simulink library "RxTxFixedPointLibrary"  (R2017b)
settings: Solver=VariableStepAuto  StartTime=0.0  StopTime=10.0  RelTol=1e-3
undefined symbols (not defined in the file): AGCBarkerSymbols, coeff, crcDecodeLag, CRCGeneratorLag, EQTrainingSymbols, j, K1, K2, numHeaderBits, numTrainingSamples, pLen, RadioSampleRate, samplesPerSymbol, VibertiTracebackLength, xPreambleSeq
libraries: simulink x27, dsphdlfiltering x20, hdlsllib x10, commseqgen3 x4, commdigbbndpm3 x3, commcrc2 x2, commcnvcod2 x2, dspsigops x2, dspstat3 x1, commfilt2 x1
(part 1 of 3)
settings Model: Creator=tcollins  LastModifiedBy=tcollins

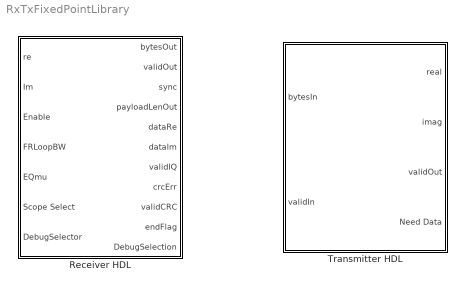
== system RxTxFixedPointLibrary ==
  Receiver HDL : Subsystem  TreatAsAtomicUnit=on
      mask Display:
      | if ispc
      |     d = '\';
      | else
      |     d = '/';
      | end
      | model_path = get_param(bdroot, 'FileName');
      | %info = Simulink.MDLInfo(bdroot)
      | c = strsplit(model_path,d); c = strjoin(c(1:end-2),d);
      | logo = [c,d,'ADI_logo.svg'];
      | %disp(logo);
      | image(logo);
  Transmitter HDL : Subsystem  TreatAsAtomicUnit=on
      mask Display:
      | if ispc
      |     d = '\';
      | else
      |     d = '/';
      | end
      | model_path = get_param(bdroot, 'FileName');
      | %info = Simulink.MDLInfo(bdroot)
      | c = strsplit(model_path,d); c = strjoin(c(1:end-2),d);
      | logo = [c,d,'ADI_logo.svg'];
      | %disp(logo);
      | image(logo);

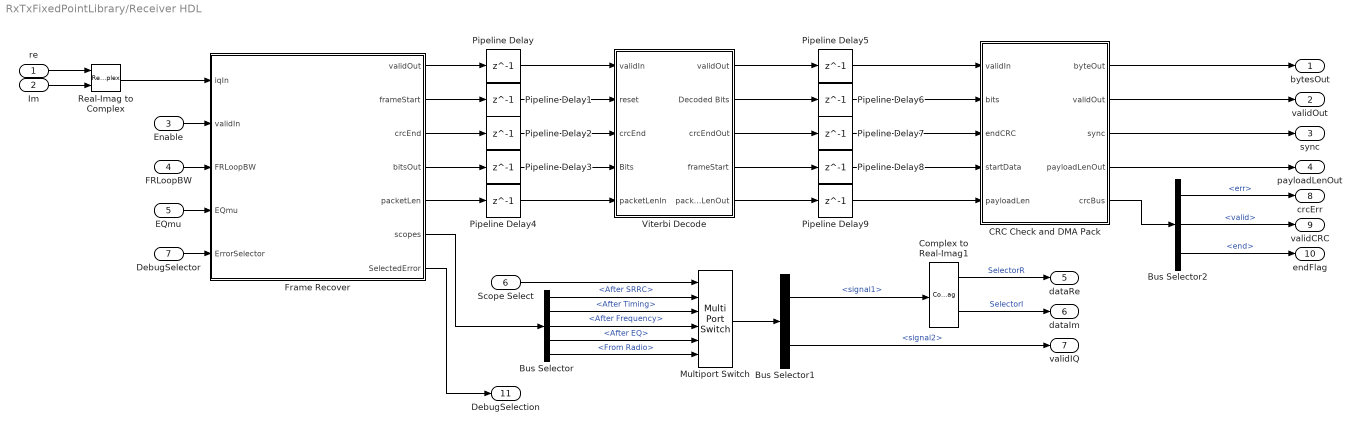
== system RxTxFixedPointLibrary/Receiver HDL ==
  re : Inport  OutDataTypeStr=int16
  Im : Inport  Port=2  OutDataTypeStr=int16
  Enable : Inport  Port=3
  FRLoopBW : Inport  Port=4
  EQmu : Inport  Port=5
  Scope Select : Inport  Port=6
  DebugSelector : Inport  Port=7
  Bus Selector : BusSelector  OutputSignals=After SRRC,After Timing,After Frequency,After EQ,From Radio
  Bus Selector1 : BusSelector  OutputSignals=signal1,signal2
  Bus Selector2 : BusSelector  OutputSignals=err,valid,end
  CRC Check and DMA Pack : Subsystem
  Complex to Real-Imag1 : ComplexToRealImag
  Frame Recover : Subsystem
  Multiport Switch : MultiPortSwitch  Inputs=5
  Pipeline Delay{,1..9} (10 alike) : Delay  DelayLength=1
  Real-Imag to Complex : RealImagToComplex
  Viterbi Decode : Subsystem  TreatAsAtomicUnit=on
  bytesOut : Outport
  validOut : Outport  Port=2
  sync : Outport  Port=3
  payloadLenOut : Outport  Port=4
  dataRe : Outport  Port=5
  dataIm : Outport  Port=6
  validIQ : Outport  Port=7
  crcErr : Outport  Port=8
  validCRC : Outport  Port=9
  endFlag : Outport  Port=10
  DebugSelection : Outport  Port=11
  wires:
  Bus Selector/5 -> Multiport Switch/6  "<From Radio>"
  Pipeline Delay5/1 -> CRC Check and DMA Pack/1(validIn)
  Bus Selector1/2 -> validIQ/1  "<signal2>"
  Bus Selector1/1 -> Complex to Real-Imag1/1  "<signal1>"
  Bus Selector/4 -> Multiport Switch/5  "<After EQ>"
  Multiport Switch/1 -> Bus Selector1/1
  Scope Select/1 -> Multiport Switch/1
  Bus Selector/2 -> Multiport Switch/3  "<After Timing>"
  Bus Selector/3 -> Multiport Switch/4  "<After Frequency>"
  Bus Selector/1 -> Multiport Switch/2  "<After SRRC>"
  Frame Recover/6(scopes) -> Bus Selector/1
  EQmu/1 -> Frame Recover/4(EQmu)
  FRLoopBW/1 -> Frame Recover/3(FRLoopBW)
  Viterbi Decode/1(validOut) -> Pipeline Delay5/1
  Pipeline Delay/1 -> Viterbi Decode/1(validIn)
  CRC Check and DMA Pack/4(payloadLenOut) -> payloadLenOut/1
  Viterbi Decode/2(Decoded Bits) -> Pipeline Delay6/1
  Pipeline Delay2/1 -> Viterbi Decode/3(crcEnd)
  CRC Check and DMA Pack/3(sync) -> sync/1
  Pipeline Delay7/1 -> CRC Check and DMA Pack/3(endCRC)
  Pipeline Delay9/1 -> CRC Check and DMA Pack/5(payloadLen)
  Pipeline Delay6/1 -> CRC Check and DMA Pack/2(bits)
  Pipeline Delay8/1 -> CRC Check and DMA Pack/4(startData)
  Pipeline Delay4/1 -> Viterbi Decode/5(packetLenIn)
  Pipeline Delay3/1 -> Viterbi Decode/4(Bits)
  Pipeline Delay1/1 -> Viterbi Decode/2(reset)
  CRC Check and DMA Pack/2(validOut) -> validOut/1
  CRC Check and DMA Pack/1(byteOut) -> bytesOut/1
  Viterbi Decode/5(packetLenOut) -> Pipeline Delay9/1
  Viterbi Decode/4(frameStart) -> Pipeline Delay8/1
  Viterbi Decode/3(crcEndOut) -> Pipeline Delay7/1
  Frame Recover/4(bitsOut) -> Pipeline Delay3/1
  Frame Recover/3(crcEnd) -> Pipeline Delay2/1
  Frame Recover/2(frameStart) -> Pipeline Delay1/1
  Frame Recover/1(validOut) -> Pipeline Delay/1
  Frame Recover/5(packetLen) -> Pipeline Delay4/1
  Complex to Real-Imag1/1 -> dataRe/1  "SelectorR"
  Complex to Real-Imag1/2 -> dataIm/1  "SelectorI"
  Im/1 -> Real-Imag to Complex/2
  re/1 -> Real-Imag to Complex/1
  CRC Check and DMA Pack/5(crcBus) -> Bus Selector2/1
  Bus Selector2/1 -> crcErr/1  "<err>"
  Bus Selector2/2 -> validCRC/1  "<valid>"
  Bus Selector2/3 -> endFlag/1  "<end>"
  Enable/1 -> Frame Recover/2(validIn)
  Real-Imag to Complex/1 -> Frame Recover/1(iqIn)
  DebugSelector/1 -> Frame Recover/5(ErrorSelector)
  Frame Recover/7(SelectedError) -> DebugSelection/1

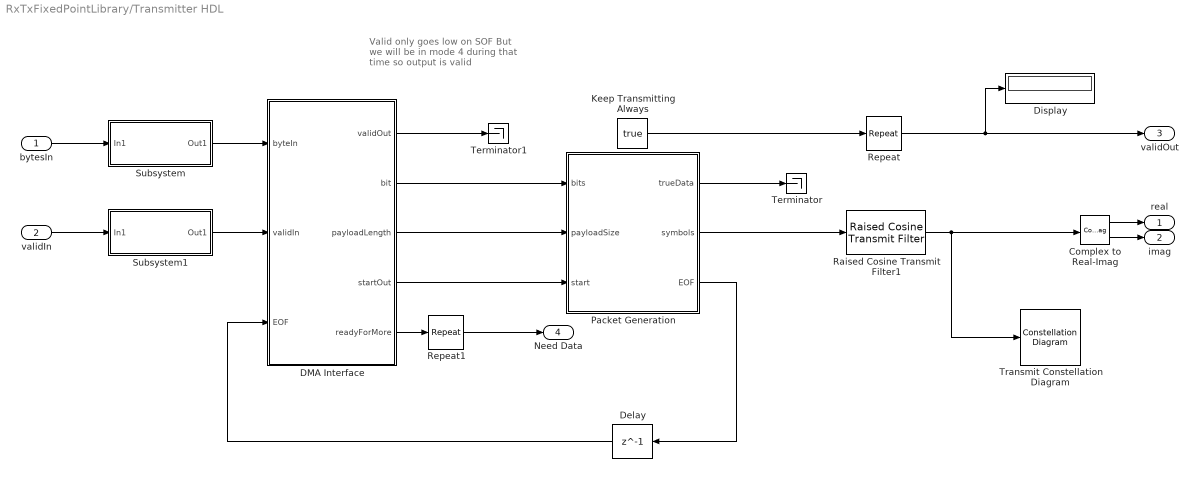
== system RxTxFixedPointLibrary/Transmitter HDL ==
  note: Valid only goes low on SOF
      | But we will be in mode 4 during
      | that time so output is valid
  bytesIn : Inport
  validIn : Inport  Port=2
  Complex to Real-Imag : ComplexToRealImag
  DMA Interface : Subsystem
  Delay : Delay  DelayLength=1
  Display : Display
  Keep Transmitting Always : Constant  Value=true  SampleTime=-1
  Packet Generation : Subsystem
  Raised Cosine Transmit Filter1 : commfilt2/Raised Cosine Transmit Filter  filtType=Square root  R=0.5  filtSpan=8  N=4  filterGain=1  RateOptions=Allow multirate processing  framing=Mute  checkCoeff=off  variableName=rcTxFilt1  checkGain=Normalized  sampMode=Mute  saveAsFlag=0  currentFiltSpan=8  D=(8)/2  launchFVT=on  roundingMode=Floor  overflowMode=off  coeffDataTypeStr=Inherit: Same word length as input  coeffMin=[]  coeffMax=[]  coeffLastDataTypeStr=Inherit: Same word length as input  outputMode=Binary point scaling  outputWordLength=16  outputFracLength=14  outputDataTypeStr=fixdt(1,16,14)  outputMin=[]  outputMax=[]  outputLastDataTypeStr=fixdt(1,16,14)
  Repeat : dspsigops/Repeat  N=4  InputProcessing=Columns as channels (frame based)  RateOptions=Allow multirate processing  ic=0  mode=Unused parameter value
      settings: SourceProductName=DSP System Toolbox
  Repeat1 : dspsigops/Repeat  N=4  InputProcessing=Columns as channels (frame based)  RateOptions=Allow multirate processing  ic=0  mode=Unused parameter value
      settings: SourceProductName=DSP System Toolbox
  Subsystem : Subsystem
  Subsystem1 : Subsystem
  Terminator : Terminator
  Terminator1 : Terminator
  Transmit Constellation Diagram : ConstellationDiagram
  real : Outport  PortDimensions=1
  imag : Outport  Port=2  PortDimensions=1
  validOut : Outport  Port=3  PortDimensions=1
  Need Data : Outport  Port=4
  wires:
  Complex to Real-Imag/1 -> real/1
  Complex to Real-Imag/2 -> imag/1
  DMA Interface/2(bit) -> Packet Generation/1(bits)
  DMA Interface/3(payloadLength) -> Packet Generation/2(payloadSize)
  DMA Interface/4(startOut) -> Packet Generation/3(start)
  Packet Generation/2(symbols) -> Raised Cosine Transmit Filter1/1
  DMA Interface/5(readyForMore) -> Repeat1/1
  Packet Generation/1(trueData) -> Terminator/1
  Packet Generation/3(EOF) -> Delay/1
  Delay/1 -> DMA Interface/3(EOF)
  bytesIn/1 -> Subsystem/1(In1)
  Repeat1/1 -> Need Data/1
  Subsystem/1(Out1) -> DMA Interface/1(byteIn)
  Subsystem1/1(Out1) -> DMA Interface/2(validIn)
  DMA Interface/1(validOut) -> Terminator1/1
  Keep Transmitting Always/1 -> Repeat/1
  validIn/1 -> Subsystem1/1(In1)
  Repeat/1 -> validOut/1, Display/1
  Raised Cosine Transmit Filter1/1 -> Transmit Constellation Diagram/1, Complex to Real-Imag/1

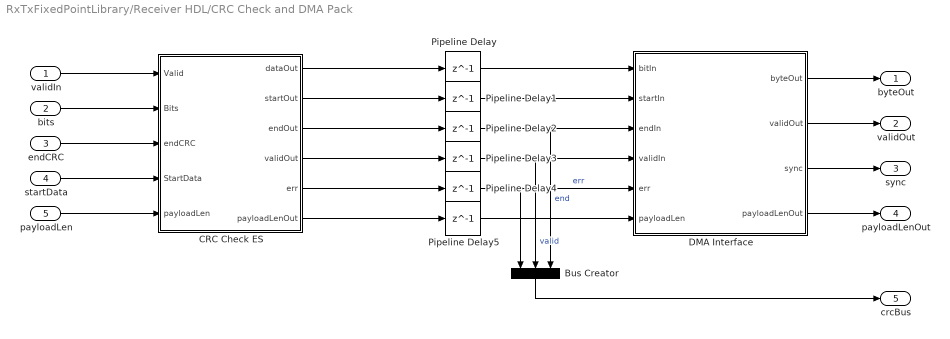
== system RxTxFixedPointLibrary/Receiver HDL/CRC Check and DMA Pack ==
  validIn : Inport  PortDimensions=1
  bits : Inport  Port=2  PortDimensions=1
  endCRC : Inport  Port=3  PortDimensions=1
  startData : Inport  Port=4  PortDimensions=1
  payloadLen : Inport  Port=5  PortDimensions=1
  Bus Creator : BusCreator  Inputs=3
  CRC Check ES : Subsystem
  DMA Interface : Subsystem
  Pipeline Delay{,1..5} (6 alike) : Delay  DelayLength=1
  byteOut : Outport
  validOut : Outport  Port=2
  sync : Outport  Port=3
  payloadLenOut : Outport  Port=4
  crcBus : Outport  Port=5
  wires:
  CRC Check ES/4(validOut) -> Pipeline Delay3/1
  DMA Interface/4(payloadLenOut) -> payloadLenOut/1
  validIn/1 -> CRC Check ES/1(Valid)
  Pipeline Delay5/1 -> DMA Interface/6(payloadLen)
  Pipeline Delay4/1 -> Bus Creator/1, DMA Interface/5(err)  "err"
  Pipeline Delay3/1 -> Bus Creator/2, DMA Interface/4(validIn)  "valid"
  Pipeline Delay2/1 -> Bus Creator/3, DMA Interface/3(endIn)  "end"
  Pipeline Delay1/1 -> DMA Interface/2(startIn)
  Pipeline Delay/1 -> DMA Interface/1(bitIn)
  endCRC/1 -> CRC Check ES/3(endCRC)
  CRC Check ES/6(payloadLenOut) -> Pipeline Delay5/1
  startData/1 -> CRC Check ES/4(StartData)
  payloadLen/1 -> CRC Check ES/5(payloadLen)
  DMA Interface/3(sync) -> sync/1
  bits/1 -> CRC Check ES/2(Bits)
  CRC Check ES/5(err) -> Pipeline Delay4/1
  CRC Check ES/1(dataOut) -> Pipeline Delay/1
  CRC Check ES/2(startOut) -> Pipeline Delay1/1
  DMA Interface/1(byteOut) -> byteOut/1
  CRC Check ES/3(endOut) -> Pipeline Delay2/1
  DMA Interface/2(validOut) -> validOut/1
  Bus Creator/1 -> crcBus/1

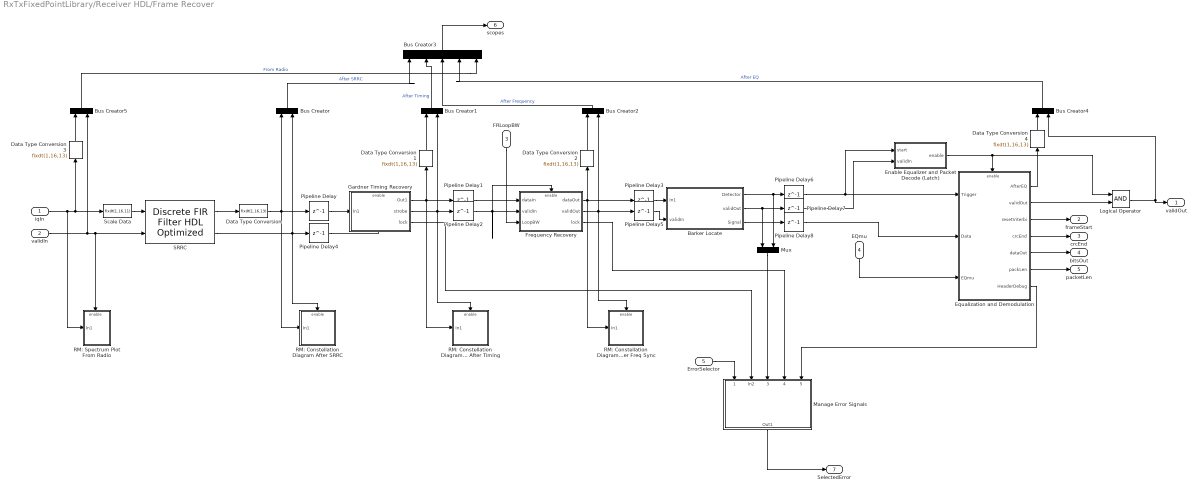
== system RxTxFixedPointLibrary/Receiver HDL/Frame Recover ==
  iqIn : Inport  PortDimensions=1
  validIn : Inport  Port=2  PortDimensions=1
  FRLoopBW : Inport  Port=3
  EQmu : Inport  Port=4
  ErrorSelector : Inport  Port=5  PortDimensions=1
  Barker Locate : Subsystem  mask{Threshold=1}
  Bus Creator{,1..2,4..5} (5 alike) : BusCreator  Inputs=2
  Bus Creator3 : BusCreator  Inputs=5
  Data Type Conversion{,1..4} (5 alike) : DataTypeConversion  OutDataTypeStr=fixdt(1,16,13)
  Enable Equalizer and Packet Decode (Latch) : MATLAB Function  TreatAsAtomicUnit=on
  Equalization and Demodulation : Subsystem
  Frequency Recovery : Subsystem
  Gardner Timing Recovery : Subsystem
  Logical Operator : Logic  AllPortsSameDT=off  OutDataTypeStr=boolean
  Manage Error Signals : Subsystem
  Mux : Mux  Inputs=2
  Pipeline Delay{,1..8} (9 alike) : Delay  DelayLength=1
  RM: Constellation Diagram After Freq Sync : Subsystem
  RM: Constellation Diagram After SRRC : Subsystem
  RM: Constellation Diagram After Timing : Subsystem
  RM: Spectrum Plot From Radio : Subsystem
  SRRC : dsphdlfiltering/Discrete FIR Filter HDL Optimized  Numerator=coeff  Sharing=off  SharingFactor=2  SimulateUsing=Code generation  roundingMode=Floor  overflowMode=on  CoefficientsDataTypeStr=Inherit: Same word length as input  CoefficientsMin=[]  CoefficientsMax=[]  OutputDataTypeStr=fixdt(1,16,11)  OutputMin=[]  OutputMax=[]  ValidInPort=on  ReadyPort=off
      settings: SourceProductName=DSP System Toolbox  SourceProductBaseCode=DS
  Scale Data : DataTypeConversion  OutDataTypeStr=fixdt(1,16,11)  ConvertRealWorld=Stored Integer (SI)  SaturateOnIntegerOverflow=on
  validOut : Outport
  frameStart : Outport  Port=2
  crcEnd : Outport  Port=3
  bitsOut : Outport  Port=4
  packetLen : Outport  Port=5
  scopes : Outport  Port=6
  SelectedError : Outport  Port=7
  wires:
  Data Type Conversion3/1 -> Bus Creator5/1
  Bus Creator5/1 -> Bus Creator3/5  "From Radio"
  Data Type Conversion4/1 -> Bus Creator4/1
  Data Type Conversion2/1 -> Bus Creator2/1
  Data Type Conversion1/1 -> Bus Creator1/1
  Bus Creator4/1 -> Bus Creator3/4  "After EQ"
  Bus Creator3/1 -> scopes/1
  Bus Creator2/1 -> Bus Creator3/3  "After Frequency"
  Bus Creator1/1 -> Bus Creator3/2  "After Timing"
  Bus Creator/1 -> Bus Creator3/1  "After SRRC"
  Frequency Recovery/2(validOut) -> RM: Constellation Diagram After Freq Sync/Enable, Bus Creator2/2, Pipeline Delay5/1
  Frequency Recovery/1(dataOut) -> Data Type Conversion2/1, RM: Constellation Diagram After Freq Sync/1(In1), Pipeline Delay3/1
  Gardner Timing Recovery/1(Out1) -> Pipeline Delay1/1, Data Type Conversion1/1, RM: Constellation Diagram After Timing/1(In1)
  Gardner Timing Recovery/2(strobe) -> RM: Constellation Diagram After Timing/Enable, Pipeline Delay2/1, Bus Creator1/2
  EQmu/1 -> Equalization and Demodulation/3(EQmu)
  FRLoopBW/1 -> Frequency Recovery/3(LoopBW)
  Pipeline Delay4/1 -> Gardner Timing Recovery/Enable
  Pipeline Delay/1 -> Gardner Timing Recovery/1(In1)
  Data Type Conversion/1 -> Bus Creator/1, Pipeline Delay/1, RM: Constellation Diagram After SRRC/1(In1)
  Logical Operator/1 -> validOut/1, Bus Creator4/2
  Pipeline Delay8/1 -> Equalization and Demodulation/2(Data)
  Pipeline Delay7/1 -> Enable Equalizer and Packet Decode (Latch)/2(validIn)
  Pipeline Delay6/1 -> Equalization and Demodulation/1(Trigger), Enable Equalizer and Packet Decode (Latch)/1(start)
  Pipeline Delay5/1 -> Barker Locate/2(validIn)
  Pipeline Delay3/1 -> Barker Locate/1(In1)
  Pipeline Delay2/1 -> Frequency Recovery/Enable, Frequency Recovery/2(validIn)
  Pipeline Delay1/1 -> Frequency Recovery/1(dataIn)
  Equalization and Demodulation/1(AfterEQ) -> Data Type Conversion4/1
  Barker Locate/1(Detector) -> Mux/2, Pipeline Delay6/1
  Equalization and Demodulation/6(packLen) -> packetLen/1
  Scale Data/1 -> SRRC/1
  Equalization and Demodulation/2(validOut) -> Logical Operator/2
  Barker Locate/3(Signal) -> Pipeline Delay8/1
  validIn/1 -> Bus Creator5/2, RM: Spectrum Plot From Radio/Enable, SRRC/2
  iqIn/1 -> RM: Spectrum Plot From Radio/1(In1), Data Type Conversion3/1, Scale Data/1
  SRRC/1 -> Data Type Conversion/1
  SRRC/2 -> Bus Creator/2, Pipeline Delay4/1, RM: Constellation Diagram After SRRC/Enable
  Equalization and Demodulation/5(dataOut) -> bitsOut/1
  Enable Equalizer and Packet Decode (Latch)/1(enable) -> Equalization and Demodulation/Enable, Logical Operator/1
  Equalization and Demodulation/4(crcEnd) -> crcEnd/1
  Barker Locate/2(validOut) -> Mux/1, Pipeline Delay7/1
  Equalization and Demodulation/3(resetViterbi) -> frameStart/1
  Mux/1 -> Manage Error Signals/3(Peak Detector)
  Frequency Recovery/3(lock) -> Manage Error Signals/4(FreqPLL Lock)
  Equalization and Demodulation/7(HeaderDebug) -> Manage Error Signals/5(Header Debug)
  Manage Error Signals/1(Out1) -> SelectedError/1
  Gardner Timing Recovery/3(lock) -> Manage Error Signals/2(In2)
  ErrorSelector/1 -> Manage Error Signals/1(ErrorSelector)

== system RxTxFixedPointLibrary/Receiver HDL/Viterbi Decode ==
  validIn : Inport
  reset : Inport  Port=2
  crcEnd : Inport  Port=3
  Bits : Inport  Port=4
  packetLenIn : Inport  Port=5
  Align with post reset data : Delay  DelayLength=1
  Buffer : Subsystem
  Logical Operator : Logic  AllPortsSameDT=off  OutDataTypeStr=boolean
  Viterbi Decoder : commcnvcod2/Viterbi Decoder  trellis=poly2trellis(7, [171 133])  isPunctured=off  punctureVector=[1; 1; 0; 1; 0; 1]  erasures=off  dectype=Hard decision  nsdecb=4  runSigValErrCheck=off  tbdepth=VibertiTracebackLength  opmode=Continuous  reset=on  delayedResetAction=on  smWordLength=16  outDataType=boolean
      settings: SourceProductName=Communications System Toolbox  SourceProductBaseCode=CM
  Viterbi Lag{,1..3} (4 alike) : Delay  DelayLength=VibertiTracebackLength
  validOut : Outport  InitialOutput=0
  Decoded Bits : Outport  Port=2  InitialOutput=0
  crcEndOut : Outport  Port=3  InitialOutput=0
  frameStart : Outport  Port=4  InitialOutput=0
  packetLenOut : Outport  Port=5  InitialOutput=0
  wires:
  Buffer/4(crcOut) -> Viterbi Lag1/1
  Viterbi Decoder/1 -> Logical Operator/1
  Logical Operator/1 -> Decoded Bits/1
  Align with post reset data/1 -> Viterbi Lag2/1
  Buffer/5(packetLenOut) -> Viterbi Lag3/1
  Viterbi Lag/1 -> validOut/1, Logical Operator/2
  Viterbi Lag1/1 -> crcEndOut/1
  Buffer/3(validOut) -> Viterbi Lag/1
  Buffer/2(resetOut) -> Viterbi Decoder/2, Align with post reset data/1
  Buffer/1(dataOut) -> Viterbi Decoder/1
  crcEnd/1 -> Buffer/4(crc)
  validIn/1 -> Buffer/3(valid)
  reset/1 -> Buffer/2(start)
  Bits/1 -> Buffer/1(data)
  Viterbi Lag2/1 -> frameStart/1
  packetLenIn/1 -> Buffer/5(packetLen)
  Viterbi Lag3/1 -> packetLenOut/1

== system RxTxFixedPointLibrary/Transmitter HDL/DMA Interface ==
  byteIn : Inport
  validIn : Inport  Port=2
  EOF : Inport  Port=3
  Align with data : Delay  DelayLength=1
  DMA Control : MATLAB Function  TreatAsAtomicUnit=on
  validOut : Outport
  bit : Outport  Port=2
  payloadLength : Outport  Port=3  OutDataTypeStr=uint16
  startOut : Outport  Port=4
  readyForMore : Outport  Port=5
  wires:
  byteIn/1 -> DMA Control/1(byteIn)
  DMA Control/1(bitOut) -> bit/1
  DMA Control/5(readyForInput) -> readyForMore/1
  DMA Control/4(payloadLength) -> payloadLength/1
  DMA Control/2(validOut) -> validOut/1
  validIn/1 -> DMA Control/2(validIn)
  Align with data/1 -> startOut/1
  DMA Control/3(startOut) -> Align with data/1
  EOF/1 -> DMA Control/3(EOF)

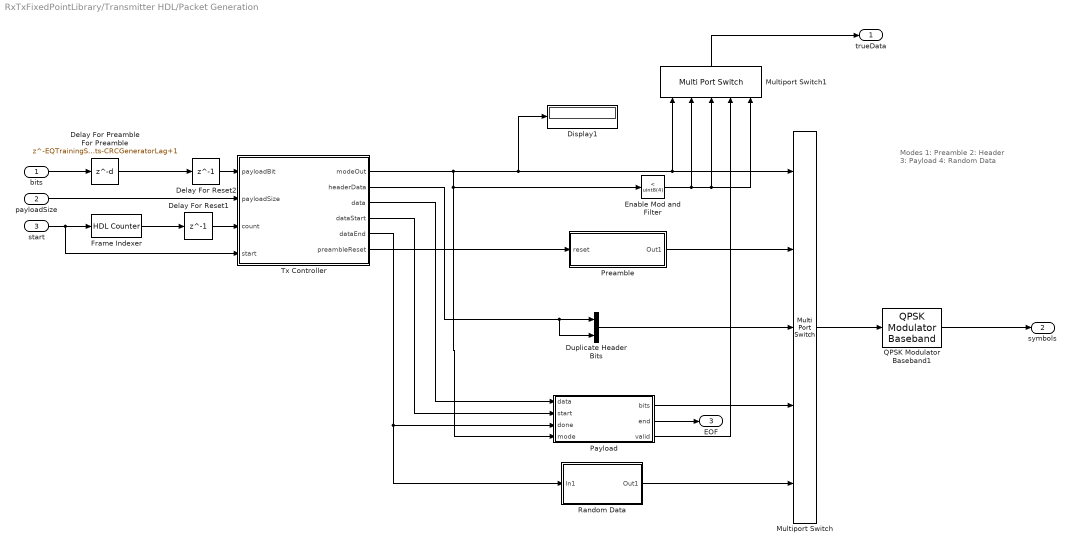
== system RxTxFixedPointLibrary/Transmitter HDL/Packet Generation ==
  note: Modes
      | 	1: Preamble
      | 	2: Header
      | 	3: Payload
      | 	4: Random Data
  bits : Inport  OutDataTypeStr=boolean
  payloadSize : Inport  Port=2
  start : Inport  Port=3
  Delay For Preamble For Preamble : Delay  DelayLength=EQTrainingSymbols+AGCBarkerSymbols+numHeaderBits-CRCGeneratorLag+1  InitialCondition=false
  Delay For Reset1 : Delay  DelayLength=1
  Delay For Reset2 : Delay  DelayLength=1  InitialCondition=false
  Display1 : Display
  Duplicate Header Bits : Concatenate
  Enable Mod and Filter : simulink/Logic and Bit Operations/Compare To Constant  relop=<  const=uint8(4)  OutDataTypeStr=boolean
  Frame Indexer : hdlsllib/Sources/HDL Counter  CountType=Count limited  CountInit=0  CountStep=1  CountMax=2^16+EQTrainingSymbols+AGCBarkerSymbols+numHeaderBits  CountFromType=Specify  CountFrom=0  CountResetPort=on  CountLoadPort=off  CountEnbPort=off  CountDirPort=off  CountDataType=Unsigned  CountWordLen=32  CountFracLen=0  CountSampTime=1
      settings: SourceProductBaseCode=HD
  Multiport Switch : MultiPortSwitch  Inputs=4
  Multiport Switch1 : MultiPortSwitch  Inputs=4
  Payload : Subsystem
  Preamble : Subsystem
  QPSK Modulator Baseband1 : commdigbbndpm3/QPSK Modulator Baseband  InType=Bit  Enc=Binary  Ph=pi/4  outDtype=Fixed-point  outWordLen=16  outUDDataType=sfix(16)  outFracLenMode=User-defined  outFracLen=15  outDataTypeStr=fixdt(1,16,15)  outLastDataTypeStr=fixdt(1,16,15)
  Random Data : Subsystem
  Tx Controller : MATLAB Function  TreatAsAtomicUnit=on
  trueData : Outport  InitialOutput=0
  symbols : Outport  Port=2  InitialOutput=complex(0)
  EOF : Outport  Port=3  OutDataTypeStr=boolean  InitialOutput=0
  wires:
  Tx Controller/2(headerData) -> Duplicate Header Bits/2, Duplicate Header Bits/1
  Random Data/1(Out1) -> Multiport Switch/5
  Enable Mod and Filter/1 -> Multiport Switch1/5, Multiport Switch1/3, Multiport Switch1/2
  Tx Controller/3(data) -> Payload/1(data)
  Tx Controller/4(dataStart) -> Payload/2(start)
  Delay For Preamble For Preamble/1 -> Delay For Reset2/1
  start/1 -> Tx Controller/4(start), Frame Indexer/1
  Preamble/1(Out1) -> Multiport Switch/2
  bits/1 -> Delay For Preamble For Preamble/1
  QPSK Modulator Baseband1/1 -> symbols/1
  Multiport Switch1/1 -> trueData/1
  Delay For Reset1/1 -> Tx Controller/3(count)
  Multiport Switch/1 -> QPSK Modulator Baseband1/1
  Tx Controller/5(dataEnd) -> Payload/3(done), Random Data/1(In1)
  Payload/1(bits) -> Multiport Switch/4
  Duplicate Header Bits/1 -> Multiport Switch/3
  Frame Indexer/1 -> Delay For Reset1/1
  Payload/3(valid) -> Multiport Switch1/4
  Payload/2(end) -> EOF/1
  payloadSize/1 -> Tx Controller/2(payloadSize)
  Tx Controller/1(modeOut) -> Display1/1, Multiport Switch/1, Multiport Switch1/1, Payload/4(mode), Enable Mod and Filter/1
  Tx Controller/6(preambleReset) -> Preamble/1(reset)
  Delay For Reset2/1 -> Tx Controller/1(payloadBit)

== system RxTxFixedPointLibrary/Transmitter HDL/Subsystem ==
  In1 : Inport
  Downsample5 : DownSample  N=4  RateOptions=Allow multirate processing
  Sum of Elements : Sum  Inputs=+  AccumDataTypeStr=fixdt(0,64,0)
  Tapped Delay : simulink/Discrete/Tapped Delay  vinit=0.0  samptime=-1  NumDelays=3  DelayOrder=Oldest  includeCurrent=on
  Out1 : Outport
  wires:
  In1/1 -> Tapped Delay/1
  Tapped Delay/1 -> Downsample5/1
  Downsample5/1 -> Sum of Elements/1
  Sum of Elements/1 -> Out1/1

== system RxTxFixedPointLibrary/Transmitter HDL/Subsystem1 ==
  In1 : Inport
  Downsample5 : DownSample  N=4  RateOptions=Allow multirate processing
  Logical Operator : Logic  Operator=OR  Inputs=1  AllPortsSameDT=off  OutDataTypeStr=boolean
  Tapped Delay : simulink/Discrete/Tapped Delay  vinit=0.0  samptime=-1  NumDelays=3  DelayOrder=Oldest  includeCurrent=on
  Out1 : Outport
  wires:
  In1/1 -> Tapped Delay/1
  Tapped Delay/1 -> Downsample5/1
  Downsample5/1 -> Logical Operator/1
  Logical Operator/1 -> Out1/1

== system RxTxFixedPointLibrary/Receiver HDL/CRC Check and DMA Pack/CRC Check ES ==
  note: NOTE:
      | 	The Valid signal must be latched during a packet, which is
      | 	a bug (2018a Fixed).
  Valid : Inport
  Bits : Inport  Port=2
  endCRC : Inport  Port=3
  StartData : Inport  Port=4
  payloadLen : Inport  Port=5
  CRC Decode Lag : Delay  DelayLength=crcDecodeLag
  Convert To fi : DataTypeConversion  OutDataTypeStr=fixdt(0,1,0)  SaturateOnIntegerOverflow=on
  DEBUG: CRC Input : MATLAB Function  Commented=on  TreatAsAtomicUnit=on
  DEBUG: Check CRC Result : MATLAB Function  Commented=on  TreatAsAtomicUnit=on
  General CRC Syndrom Detector HDL Optimized : commcrc2/General CRC Syndrome Detector HDL Optimized  Polynomial=crc32Poly  InitialState=0  DirectMethod=off  ReflectInput=off  ReflectCRCChecksum=off  FinalXORValue=0  SimulateUsing=Code generation
      settings: SourceProductName=Communications System Toolbox  SourceProductBaseCode=CM
  dataOut : Outport  InitialOutput=0
  startOut : Outport  Port=2  InitialOutput=0
  endOut : Outport  Port=3  InitialOutput=0
  validOut : Outport  Port=4  InitialOutput=0
  err : Outport  Port=5  InitialOutput=0
  payloadLenOut : Outport  Port=6  InitialOutput=0
  wires:
  Valid/1 -> DEBUG: CRC Input/2(enable), General CRC Syndrom Detector HDL Optimized/4
  endCRC/1 -> General CRC Syndrom Detector HDL Optimized/3, DEBUG: CRC Input/3(endFlag)
  StartData/1 -> General CRC Syndrom Detector HDL Optimized/2, DEBUG: CRC Input/4(startFlag)
  CRC Decode Lag/1 -> payloadLenOut/1
  payloadLen/1 -> CRC Decode Lag/1
  Convert To fi/1 -> General CRC Syndrom Detector HDL Optimized/1
  General CRC Syndrom Detector HDL Optimized/2 -> startOut/1, DEBUG: Check CRC Result/2(start)
  General CRC Syndrom Detector HDL Optimized/5 -> err/1, DEBUG: Check CRC Result/5(err)
  General CRC Syndrom Detector HDL Optimized/4 -> validOut/1, DEBUG: Check CRC Result/4(valid)
  General CRC Syndrom Detector HDL Optimized/3 -> endOut/1, DEBUG: Check CRC Result/3(done)
  General CRC Syndrom Detector HDL Optimized/1 -> dataOut/1, DEBUG: Check CRC Result/1(bits)
  Bits/1 -> DEBUG: CRC Input/1(u), Convert To fi/1

== system RxTxFixedPointLibrary/Receiver HDL/CRC Check and DMA Pack/DMA Interface ==
  bitIn : Inport
  startIn : Inport  Port=2
  endIn : Inport  Port=3
  validIn : Inport  Port=4
  err : Inport  Port=5
  payloadLen : Inport  Port=6
  Bit Packer : MATLAB Function  TreatAsAtomicUnit=on
  Convert Payload Length To Bytes : Subsystem
  Data Type Conversion : DataTypeConversion  OutDataTypeStr=boolean
  Delay : Delay  DelayLength=1
  Delay Error To Last Byte of Out : Delay  DelayLength=1
  Display : Display
  byteOut : Outport
  validOut : Outport  Port=2
  sync : Outport  Port=3
  payloadLenOut : Outport  Port=4
  wires:
  Convert Payload Length To Bytes/1(packetLengthOut) -> payloadLenOut/1  "packetLenOut"
  payloadLen/1 -> Convert Payload Length To Bytes/1(In1)
  Data Type Conversion/1 -> Bit Packer/1(bitIn)
  startIn/1 -> Bit Packer/2(startIn)
  endIn/1 -> Delay/1
  validIn/1 -> Bit Packer/5(validIn)
  err/1 -> Delay Error To Last Byte of Out/1
  Bit Packer/1(byteOut) -> byteOut/1, Display/1
  Bit Packer/3(startOut) -> sync/1
  Bit Packer/2(validOut) -> validOut/1
  Delay Error To Last Byte of Out/1 -> Bit Packer/4(err)
  Delay/1 -> Bit Packer/3(endIn)
  bitIn/1 -> Data Type Conversion/1

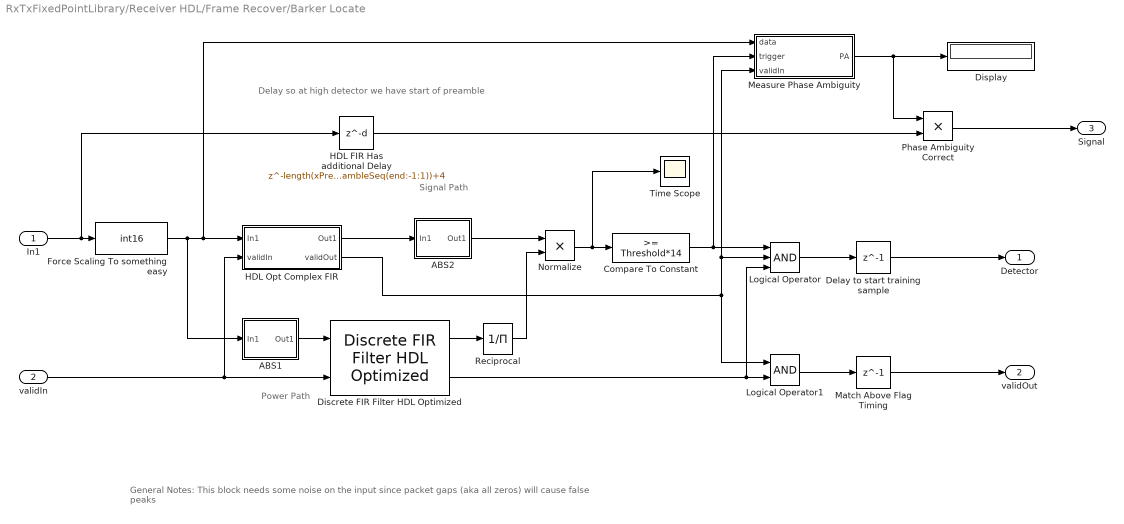
== system RxTxFixedPointLibrary/Receiver HDL/Frame Recover/Barker Locate ==
  note: Signal Path
  note: Power Path
  note: Delay so at high detector we have start of preamble
  note: General Notes:
      | This block needs some noise on the input since packet gaps (aka all zeros) will cause false peaks
  In1 : Inport  PortDimensions=1
  validIn : Inport  Port=2  PortDimensions=1
  ABS1 : Subsystem
  ABS2 : Subsystem
  Compare To Constant : simulink/Logic and Bit Operations/Compare To Constant  relop=>=  const=Threshold*14  OutDataTypeStr=boolean
  "Delay to start training sample " : Delay  DelayLength=1
  Discrete FIR Filter HDL Optimized : dsphdlfiltering/Discrete FIR Filter HDL Optimized  Numerator=ones(1,length(xPreambleSeq)*1)/1  Sharing=off  SharingFactor=2  SimulateUsing=Code generation  roundingMode=Floor  overflowMode=off  CoefficientsDataTypeStr=Inherit: Same word length as input  CoefficientsMin=[]  CoefficientsMax=[]  OutputDataTypeStr=fixdt(1,17,0)  OutputMin=[]  OutputMax=[]  ValidInPort=on  ReadyPort=off
      settings: SourceProductName=DSP System Toolbox  SourceProductBaseCode=DS
  Display : Display
  Force Scaling To something easy : DataTypeConversion  OutDataTypeStr=int16  SaturateOnIntegerOverflow=on
  HDL FIR Has additional Delay : Delay  DelayLength=length(xPreambleSeq(end:-1:1))+4
  HDL Opt Complex FIR : Subsystem  mask{Taps=xPreambleSeq(end:-1:1).'}
  Logical Operator : Logic  Inputs=3  AllPortsSameDT=off  OutDataTypeStr=boolean
  Logical Operator1 : Logic  AllPortsSameDT=off  OutDataTypeStr=boolean
  Match Above Flag Timing : Delay  DelayLength=1
  Measure Phase Ambiguity : Subsystem
  Normalize : Product  Inputs=**  OutDataTypeStr=int16  RndMeth=Simplest  SaturateOnIntegerOverflow=on
  Phase Ambiguity Correct : Product  OutDataTypeStr=fixdt(1,16,14)
  Reciprocal : Product  Inputs=/  SaturateOnIntegerOverflow=on  RndMeth=Zero
  Time Scope : Scope
  Detector : Outport
  validOut : Outport  Port=2
  Signal : Outport  Port=3
  wires:
  Match Above Flag Timing/1 -> validOut/1
  Reciprocal/1 -> Normalize/2
  Discrete FIR Filter HDL Optimized/1 -> Reciprocal/1
  Compare To Constant/1 -> Logical Operator/1, Measure Phase Ambiguity/2(trigger)
  Force Scaling To something easy/1 -> Measure Phase Ambiguity/1(data), HDL Opt Complex FIR/1(In1), ABS1/1(In1)
  HDL FIR Has additional Delay/1 -> Phase Ambiguity Correct/2
  Phase Ambiguity Correct/1 -> Signal/1
  HDL Opt Complex FIR/2(validOut) -> Logical Operator/2, Measure Phase Ambiguity/3(validIn), Logical Operator1/1
  Discrete FIR Filter HDL Optimized/2 -> Logical Operator/3, Logical Operator1/2
  validIn/1 -> Discrete FIR Filter HDL Optimized/2, HDL Opt Complex FIR/2(validIn)
  Measure Phase Ambiguity/1(PA) -> Phase Ambiguity Correct/1, Display/1
  Logical Operator1/1 -> Match Above Flag Timing/1
  Logical Operator/1 -> "Delay to start training sample "/1
  ABS1/1(Out1) -> Discrete FIR Filter HDL Optimized/1
  In1/1 -> Force Scaling To something easy/1, HDL FIR Has additional Delay/1
  Normalize/1 -> Compare To Constant/1, Time Scope/1
  "Delay to start training sample "/1 -> Detector/1
  ABS2/1(Out1) -> Normalize/1
  HDL Opt Complex FIR/1(Out1) -> ABS2/1(In1)

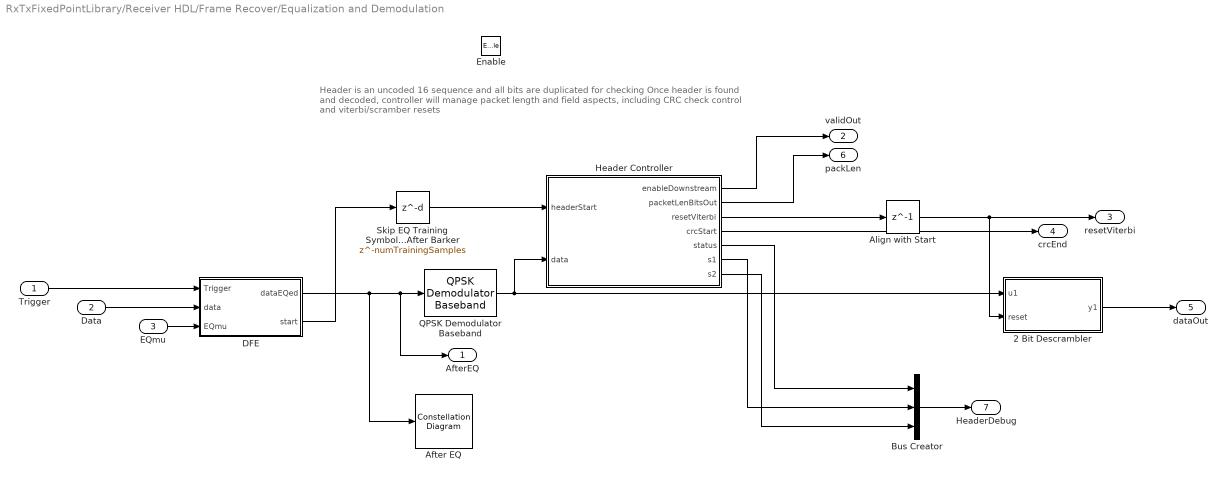
== system RxTxFixedPointLibrary/Receiver HDL/Frame Recover/Equalization and Demodulation ==
  note: Header is an uncoded 16 sequence and all bits are duplicated for checking
      |
      | Once header is found and decoded, controller will manage packet length and field aspects,
      | including CRC check control and viterbi/scramber resets
  Trigger : Inport
  Data : Inport  Port=2
  EQmu : Inport  Port=3
  Enable : EnablePort
  2 Bit Descrambler : Subsystem  mask{polynom=[1 1 0 1 0 1 0 1], initstate=[0 1 0 0 0 1 0]}
      mask prompts: polynom "Polynomial"; initstate "Inital State"
      mask Display: fprintf('HDL Descrambler')
  After EQ : ConstellationDiagram
  Align with Start : Delay  DelayLength=1
  Bus Creator : BusCreator  Inputs=3
  DFE : Subsystem
  Header Controller : MATLAB Function  TreatAsAtomicUnit=on
  QPSK Demodulator Baseband : commdigbbndpm3/QPSK Demodulator Baseband  OutType=Bit  DecType=Hard decision  VarSource=Dialog  Variance=1  Dec=Binary  Ph=pi/4  outDtype1=boolean  outDtype2=Inherit via internal rule  derotateFactorWordLen=16  derotateFactorDataTypeStr=Inherit: Same word length as input  derotateFactorLastDataTypeStr=Inherit: Same word length as input
  Skip EQ Training Symbols After Barker : Delay  DelayLength=numTrainingSamples
  AfterEQ : Outport  InitialOutput=0
  validOut : Outport  Port=2  InitialOutput=0
  resetViterbi : Outport  Port=3  InitialOutput=0
  crcEnd : Outport  Port=4  InitialOutput=0
  dataOut : Outport  Port=5  InitialOutput=0
  packLen : Outport  Port=6  InitialOutput=0
  HeaderDebug : Outport  Port=7  InitialOutput=0
  wires:
  Header Controller/1(enableDownstream) -> validOut/1
  Align with Start/1 -> resetViterbi/1, 2 Bit Descrambler/2(reset)
  Header Controller/7(s2) -> Bus Creator/3
  Header Controller/6(s1) -> Bus Creator/2
  Header Controller/5(status) -> Bus Creator/1
  EQmu/1 -> DFE/3(EQmu)
  DFE/2(start) -> Skip EQ Training Symbols After Barker/1
  Data/1 -> DFE/2(data)
  Trigger/1 -> DFE/1(Trigger)
  2 Bit Descrambler/1(y1) -> dataOut/1
  QPSK Demodulator Baseband/1 -> Header Controller/2(data), 2 Bit Descrambler/1(u1)
  Header Controller/4(crcStart) -> crcEnd/1
  Header Controller/3(resetViterbi) -> Align with Start/1
  Header Controller/2(packetLenBitsOut) -> packLen/1
  DFE/1(dataEQed) -> QPSK Demodulator Baseband/1, AfterEQ/1, After EQ/1
  Skip EQ Training Symbols After Barker/1 -> Header Controller/1(headerStart)
  Bus Creator/1 -> HeaderDebug/1

== system RxTxFixedPointLibrary/Receiver HDL/Frame Recover/Frequency Recovery ==
  note: Pull in range (Hz) = 2*pi*sqrt(2)*DampingFactor*NormLoopBandwidth*SampleRate
  note: Frequency Lock Delay = SampleRate*4*NormalizedPullInRange^2)/ (SampleRate*NormLoopBandwidth)^3;
  note: Max Phase Lock Delay= 1.3/(NormLoopBandwidth*SampleRate)
  note: Decrease Loop bandwidth to reduce phase noise,
      | but worse pull-in range
      | -0.1 30kHz pull-in
      | -0.01 5kHz pull-in
  dataIn : Inport
  validIn : Inport  Port=2
  LoopBW : Inport  Port=3
  Enable : EnablePort
  Delay : Delay  DelayLength=1
  Lock Detector : Subsystem  mask{Threshold=0.03, WindowLength=100}
      mask prompts: WindowLength "Window Length"
  Loop Filter : Subsystem  Commented=on  mask{BnTs=0.1, zeta=4*1/sqrt(2), N=1}
      mask prompts: BnTs "Normalized Loop Bandwidth"; zeta "Damping Factor"; N "Number of Samples/Symbol"
      mask init:
      | % See C.57 to C.61 in Michael Rice's "Digital Communications 
      | % - A Discrete-Time Approach" for details
      | 
      | %theta = BnTs/(zeta+0.25/zeta);  %0.0385
      | %d = 1 + 2*zeta*theta + theta*theta; %1.1938
      | %K1 = zeta*theta/d; %0.0805
      | %K2 = theta*theta/(d*2); %6.1958e-04
      | 
      | %%
      | DampingFactor = zeta;
      | samplesPerSymbol = N;
      | NormalizedLoopBandwidth = BnTs;
      | %
      | PhaseRecoveryLoopBandwidth = NormalizedLoopBandwidth*samplesPerSymbol;
      |  
      | PhaseRecoveryGain = samplesPerSymbol;
      |  
      | PhaseErrorDetectorGain = 1;
      | 
      | 
      | theta = PhaseRecoveryLoopBandwidth/...
      |     ((DampingFactor + 0.25/DampingFactor)*samplesPerSymbol);
      |  
      | d = 1 + 2*DampingFactor*theta + theta*theta;
      |  
      | % K1
      | K1 = (4*DampingFactor*theta/d)/...
      |     (PhaseErrorDetectorGain*PhaseRecoveryGain);
      | % K2
      | K2 = (4/samplesPerSymbol*theta*theta/d)/...
      |     (PhaseErrorDetectorGain*PhaseRecoveryGain);
      mask Display: disp('Loop Filter')
  Loop Filter Configurable : Subsystem
      mask Display: disp('Loop Filter')
  PED : MATLAB Function  TreatAsAtomicUnit=on
  Phase Shift FP : Subsystem
  State Control : StateControl  StateControl=Synchronous
  dataOut : Outport
  validOut : Outport  Port=2
  lock : Outport  Port=3
  wires:
  LoopBW/1 -> Loop Filter Configurable/2(LoopBW)
  validIn/1 -> validOut/1
  Phase Shift FP/1(Out1) -> Delay/1
  dataIn/1 -> Phase Shift FP/1(In1)
  Loop Filter Configurable/1(v) -> Phase Shift FP/2(Phi)
  PED/1(e) -> Loop Filter Configurable/1(e), Lock Detector/1(ped)
  Delay/1 -> dataOut/1, PED/1(In)
  Lock Detector/1(lock) -> lock/1

== system RxTxFixedPointLibrary/Receiver HDL/Frame Recover/Gardner Timing Recovery ==
  In1 : Inport
  Enable : EnablePort
  Delay : Delay  DelayLength=1
  Delay1 : Delay  DelayLength=1
  Delay2 : Delay  DelayLength=6
  Gardner TED Blocks : Subsystem
  InterpControl_Blocks1 : Subsystem
  Interpolator : Subsystem
  LoopFilter1 : Subsystem  mask{zeta=sqrt(2), BnTs=0.01, Kp=2.7}
      mask prompts: zeta "DampingFactor"; BnTs "NormalizedLoopBandwidth"; Kp "DetectionGain"
      mask init:
      | K0 = -1;
      | SPS = 4;
      | theta = BnTs/SPS/(zeta + 0.25/zeta);
      | d  = (1 + 2*zeta*theta + theta^2) * K0 * Kp;
      | ProportionalGain = (4*zeta*theta) /d;
      | IntegratorGain   = (4*theta*theta)/d;
  State Control : StateControl  StateControl=Synchronous
  TED Lock Detector : Subsystem  AncestorBlock=RxTxFixedPointLibrary/Receiver HDL/Frame Recover/Frequency Recovery/Lock Detector  mask{Threshold=0.01, WindowLength=100}
      mask prompts: WindowLength "Window Length"
  Out1 : Outport  InitialOutput=0
  strobe : Outport  Port=2  InitialOutput=false
  lock : Outport  Port=3  InitialOutput=0
  wires:
  Delay2/1 -> Interpolator/1(In1)
  LoopFilter1/1(v) -> InterpControl_Blocks1/1(e)
  InterpControl_Blocks1/2(mu) -> Delay/1
  InterpControl_Blocks1/1(strobe) -> Delay1/1
  Gardner TED Blocks/1(e) -> TED Lock Detector/1(ted), LoopFilter1/1(e)
  Interpolator/1(Out1) -> Out1/1, Gardner TED Blocks/1(data)
  Delay/1 -> Interpolator/2(mu)
  Delay1/1 -> strobe/1, Gardner TED Blocks/2(strobe)
  In1/1 -> Delay2/1
  TED Lock Detector/1(lock) -> lock/1

== system RxTxFixedPointLibrary/Receiver HDL/Frame Recover/Manage Error Signals ==
  ErrorSelector : Inport
  In2 : Inport  Port=2
  Peak Detector : Inport  Port=3
  FreqPLL Lock : Inport  Port=4
  Header Debug : Inport  Port=5
  Bus Selector : BusSelector  OutputSignals=status,s1,s2
  Compare To Constant : simulink/Logic and Bit Operations/Compare To Constant  relop===  const=uint8(2)  OutDataTypeStr=boolean
  Data Type Conversion : DataTypeConversion  OutDataTypeStr=int32
  Data Type Conversion1 : DataTypeConversion  OutDataTypeStr=int32
  Demux : Demux  Outputs=2
  Header Failure Counter : hdlsllib/Sources/HDL Counter  CountType=Count limited  CountInit=0  CountStep=1  CountMax=2^32-1  CountFromType=Initial value  CountFrom=0  CountResetPort=off  CountLoadPort=off  CountEnbPort=on  CountDirPort=off  CountDataType=Unsigned  CountWordLen=32  CountFracLen=0  CountSampTime=1
      settings: SourceProductBaseCode=HD
  Logical Operator : Logic  AllPortsSameDT=off  OutDataTypeStr=boolean
  Multiport Switch : MultiPortSwitch  Inputs=4
  Peak Detector Counter : hdlsllib/Sources/HDL Counter  CountType=Count limited  CountInit=0  CountStep=1  CountMax=2^32-1  CountFromType=Initial value  CountFrom=0  CountResetPort=off  CountLoadPort=off  CountEnbPort=on  CountDirPort=off  CountDataType=Unsigned  CountWordLen=32  CountFracLen=0  CountSampTime=1
      settings: SourceProductBaseCode=HD
  Subsystem : Subsystem
  Out1 : Outport
  wires:
  Peak Detector/1 -> Demux/1
  Demux/1 -> Subsystem/Enable, Logical Operator/1
  Demux/2 -> Logical Operator/2
  Logical Operator/1 -> Peak Detector Counter/1
  Multiport Switch/1 -> Out1/1
  ErrorSelector/1 -> Multiport Switch/1
  Header Debug/1 -> Bus Selector/1
  Bus Selector/1 -> Subsystem/1(<status>), Compare To Constant/1  "<status>"
  Compare To Constant/1 -> Header Failure Counter/1
  FreqPLL Lock/1 -> Data Type Conversion/1
  In2/1 -> Data Type Conversion1/1
  Data Type Conversion1/1 -> Multiport Switch/2
  Peak Detector Counter/1 -> Multiport Switch/3
  Data Type Conversion/1 -> Multiport Switch/4
  Header Failure Counter/1 -> Multiport Switch/5
  Bus Selector/2 -> Subsystem/2(<s1>)  "<s1>"
  Bus Selector/3 -> Subsystem/3(<s2>)  "<s2>"

== system RxTxFixedPointLibrary/Receiver HDL/Frame Recover/RM: Constellation Diagram After Freq Sync ==
  In1 : Inport
  Enable : EnablePort
  After Frequency Recovery : ConstellationDiagram
  wires:
  In1/1 -> After Frequency Recovery/1

== system RxTxFixedPointLibrary/Receiver HDL/Frame Recover/RM: Constellation Diagram After SRRC ==
  In1 : Inport
  Enable : EnablePort
  After SRRC : ConstellationDiagram
  wires:
  In1/1 -> After SRRC/1

== system RxTxFixedPointLibrary/Receiver HDL/Frame Recover/RM: Constellation Diagram After Timing ==
  In1 : Inport
  Enable : EnablePort
  After Timing Recovery : ConstellationDiagram
  wires:
  In1/1 -> After Timing Recovery/1

== system RxTxFixedPointLibrary/Receiver HDL/Frame Recover/RM: Spectrum Plot From Radio ==
  In1 : Inport
  Enable : EnablePort
  From Radio : SpectrumAnalyzer
  wires:
  In1/1 -> From Radio/1

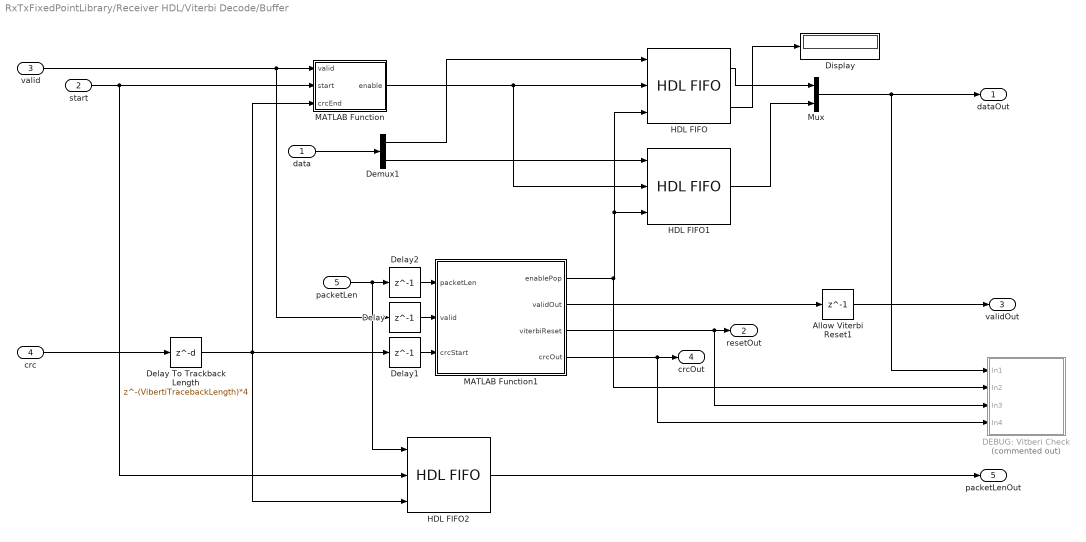
== system RxTxFixedPointLibrary/Receiver HDL/Viterbi Decode/Buffer ==
  data : Inport
  start : Inport  Port=2
  valid : Inport  Port=3
  crc : Inport  Port=4
  packetLen : Inport  Port=5
  Allow Viterbi Reset1 : Delay  DelayLength=1
  DEBUG: Vitberi Check : Subsystem  Commented=on
  Delay : Delay  DelayLength=1
  Delay To Trackback Length : Delay  DelayLength=(VibertiTracebackLength)*4
  Delay1 : Delay  DelayLength=1
  Delay2 : Delay  DelayLength=1
  Demux1 : Demux  Outputs=2
  Display : Display
  HDL FIFO : hdlsllib/HDL RAMs/HDL FIFO  fifo_size=2^16  ratio=1  push_msg=Warning  pop_msg=Warning  show_empty=off  show_full=off  show_num=on
      settings: SourceProductName=HDL Coder  SourceProductBaseCode=HD
  HDL FIFO1 : hdlsllib/HDL RAMs/HDL FIFO  fifo_size=2^16  ratio=1  push_msg=Warning  pop_msg=Warning  show_empty=off  show_full=off  show_num=off
      settings: SourceProductName=HDL Coder  SourceProductBaseCode=HD
  HDL FIFO2 : hdlsllib/HDL RAMs/HDL FIFO  fifo_size=2^3  ratio=1  push_msg=Warning  pop_msg=Warning  show_empty=off  show_full=off  show_num=off
      settings: SourceProductName=HDL Coder  SourceProductBaseCode=HD
  MATLAB Function : MATLAB Function  TreatAsAtomicUnit=on
  MATLAB Function1 : MATLAB Function  TreatAsAtomicUnit=on
  Mux : Mux  Inputs=2
  dataOut : Outport
  resetOut : Outport  Port=2
  validOut : Outport  Port=3
  crcOut : Outport  Port=4  OutDataTypeStr=boolean
  packetLenOut : Outport  Port=5
  wires:
  MATLAB Function1/3(viterbiReset) -> resetOut/1, DEBUG: Vitberi Check/3(In3)
  MATLAB Function1/4(crcOut) -> crcOut/1, DEBUG: Vitberi Check/4(In4)
  MATLAB Function1/2(validOut) -> Allow Viterbi Reset1/1
  Delay To Trackback Length/1 -> HDL FIFO2/3, MATLAB Function/3(crcEnd), Delay1/1
  Mux/1 -> dataOut/1, DEBUG: Vitberi Check/1(In1)
  crc/1 -> Delay To Trackback Length/1
  Allow Viterbi Reset1/1 -> validOut/1
  MATLAB Function1/1(enablePop) -> HDL FIFO/3, HDL FIFO1/3, DEBUG: Vitberi Check/2(In2)
  Delay2/1 -> MATLAB Function1/1(packetLen)
  Delay1/1 -> MATLAB Function1/3(crcStart)
  Delay/1 -> MATLAB Function1/2(valid)
  start/1 -> HDL FIFO2/2, MATLAB Function/2(start)
  valid/1 -> MATLAB Function/1(valid), Delay/1
  packetLen/1 -> HDL FIFO2/1, Delay2/1
  HDL FIFO2/1 -> packetLenOut/1
  HDL FIFO/2 -> Display/1
  MATLAB Function/1(enable) -> HDL FIFO/2, HDL FIFO1/2
  Demux1/2 -> HDL FIFO1/1
  HDL FIFO1/1 -> Mux/2
  HDL FIFO/1 -> Mux/1
  data/1 -> Demux1/1
  Demux1/1 -> HDL FIFO/1

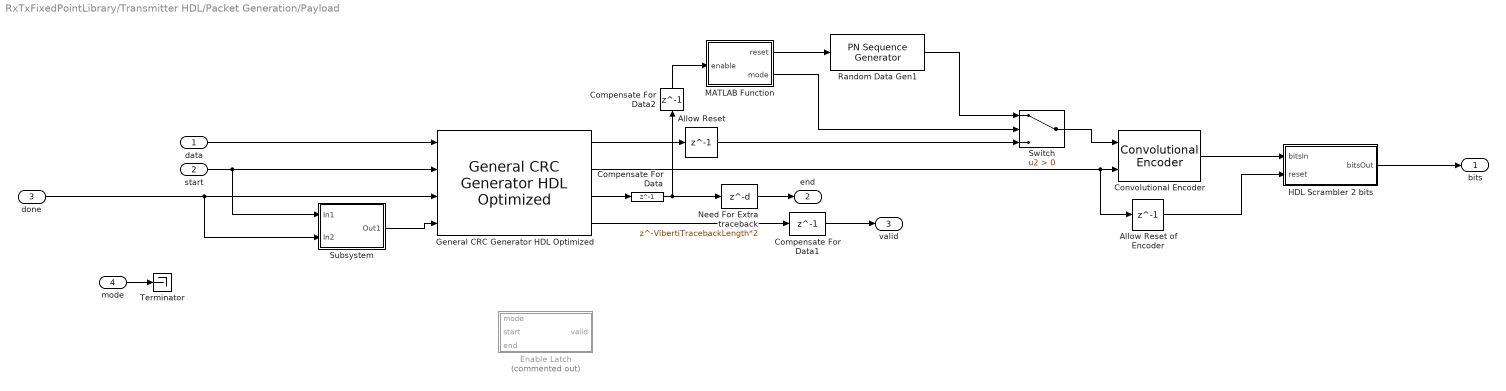
== system RxTxFixedPointLibrary/Transmitter HDL/Packet Generation/Payload ==
  data : Inport
  start : Inport  Port=2
  done : Inport  Port=3
  mode : Inport  Port=4
  Allow Reset : Delay  DelayLength=1
  Allow Reset of Encoder : Delay  DelayLength=1
  Compensate For Data : Delay  DelayLength=1
  Compensate For Data1 : Delay  DelayLength=1
  Compensate For Data2 : Delay  DelayLength=1
  Convolutional Encoder : commcnvcod2/Convolutional Encoder  trellis=poly2trellis(7, [171 133])  opMode=Reset on nonzero input via port  DelayedResetAction=on  hasIniStPort=off  hasFinStPort=off  usePuncVector=off  punctureVector=[1; 1; 0; 1; 0; 1]  reset=Unused parameter value
      settings: SourceProductName=Communications System Toolbox  SourceProductBaseCode=CM
  Enable Latch : Subsystem  Commented=on
  General CRC Generator HDL Optimized : commcrc2/General CRC Generator HDL Optimized  Polynomial=[1 0 0 0 0 0 1 0 0 1 1 0 0 0 0 0 1 0 0 0 1 1 1 0 1 1 0 1 1 0 1 1 1]  InitialState=0  DirectMethod=off  ReflectInput=off  ReflectCRCChecksum=off  FinalXORValue=0  SimulateUsing=Code generation
      settings: SourceProductName=Communications System Toolbox  SourceProductBaseCode=CM
  HDL Scrambler 2 bits : Subsystem  mask{poly=[1 1 0 1 0 1 0 1], init_state=[0 1 0 0 0 1 0]}
      mask prompts: poly "Polynomial"; init_state "Initial State"
  MATLAB Function : MATLAB Function  TreatAsAtomicUnit=on
  Need For Extra traceback : Delay  DelayLength=VibertiTracebackLength*2
  Random Data Gen1 : commseqgen3/PN Sequence Generator  poly='z^10 + z^7 + 1'  ini_sta=[0 0 1 0 0 1 0 0 1 1]  outBitMaskSource=Dialog parameter  shift=0  outVarSiz=off  maxOutSizeMode=Dialog parameter  maxOutSize=[10 1]  Ts=-1  sampPerFrame=1  reset=on  bitPackedOutputs=on  outDataType=double  numPackedBits=1  bitPackDataSigned=off  bitPackedOutDType=Smallest integer
      settings: SourceProductName=Communications System Toolbox
  Subsystem : Subsystem
  Switch : Switch  Criteria=u2 > Threshold
  Terminator : Terminator
  bits : Outport
  end : Outport  Port=2
  valid : Outport  Port=3
  wires:
  General CRC Generator HDL Optimized/1 -> Allow Reset/1
  data/1 -> General CRC Generator HDL Optimized/1
  start/1 -> Subsystem/1(In1), General CRC Generator HDL Optimized/2
  General CRC Generator HDL Optimized/4 -> Compensate For Data1/1
  mode/1 -> Terminator/1
  Convolutional Encoder/1 -> HDL Scrambler 2 bits/1(bitsIn)
  General CRC Generator HDL Optimized/2 -> Allow Reset of Encoder/1, Convolutional Encoder/2
  HDL Scrambler 2 bits/1(bitsOut) -> bits/1
  Allow Reset of Encoder/1 -> HDL Scrambler 2 bits/2(reset)
  Compensate For Data/1 -> Need For Extra traceback/1, Compensate For Data2/1
  General CRC Generator HDL Optimized/3 -> Compensate For Data/1
  MATLAB Function/1(reset) -> Random Data Gen1/1
  Switch/1 -> Convolutional Encoder/1
  Random Data Gen1/1 -> Switch/1
  Allow Reset/1 -> Switch/3
  MATLAB Function/2(mode) -> Switch/2
  Compensate For Data1/1 -> valid/1
  Need For Extra traceback/1 -> end/1
  Subsystem/1(Out1) -> General CRC Generator HDL Optimized/4
  done/1 -> Subsystem/2(In2), General CRC Generator HDL Optimized/3
  Compensate For Data2/1 -> MATLAB Function/1(enable)

== system RxTxFixedPointLibrary/Transmitter HDL/Packet Generation/Preamble ==
  reset : Inport
  Barker Even : LookupNDDirect  NumberOfTableDimensions=1  Table=[PreambleBarkersBits(4:2:end),false(1,400)]  DiagnosticForOutOfRangeInput=Error  TableDataTypeStr=boolean
  Barker Odd : LookupNDDirect  NumberOfTableDimensions=1  Table=[PreambleBarkersBits(3:2:end-1),false(1,400)]  DiagnosticForOutOfRangeInput=Error  TableDataTypeStr=boolean
  Delay{,1..3} (4 alike) : Delay  DelayLength=1
  Enable at end of barker : simulink/Logic and Bit Operations/Compare To Constant  relop=<  const=pLen/2-1  OutDataTypeStr=boolean
  HDL Counter : hdlsllib/Sources/HDL Counter  CountType=Count limited  CountInit=0  CountStep=1  CountMax=pLen/2-2+400  CountFromType=Initial value  CountFrom=0  CountResetPort=on  CountLoadPort=off  CountEnbPort=off  CountDirPort=off  CountDataType=Unsigned  CountWordLen=16  CountFracLen=0  CountSampTime=1
      settings: SourceProductBaseCode=HD
  PN Sequence For EQ : commseqgen3/PN Sequence Generator  poly='z^5 + z^3 + z^1 + 1'  ini_sta=[1 1 1 0 0]  outBitMaskSource=Dialog parameter  shift=0  outVarSiz=off  maxOutSizeMode=Dialog parameter  maxOutSize=[10 1]  Ts=-1  sampPerFrame=1  reset=on  bitPackedOutputs=on  outDataType=double  numPackedBits=2  bitPackDataSigned=off  bitPackedOutDType=Smallest integer
      settings: SourceProductName=Communications System Toolbox
  Reset When Barkers Are Done : simulink/Logic and Bit Operations/Compare To Constant  relop===  const=pLen/2-1  OutDataTypeStr=boolean
  Switch1 : Switch  Threshold=1
  Unpack1 : Subsystem
  Vector Concatenate1 : Concatenate
  Out1 : Outport
  wires:
  reset/1 -> HDL Counter/1
  Barker Odd/1 -> Vector Concatenate1/1
  Barker Even/1 -> Vector Concatenate1/2
  PN Sequence For EQ/1 -> Unpack1/1(In1)
  Switch1/1 -> Out1/1
  Reset When Barkers Are Done/1 -> PN Sequence For EQ/1
  HDL Counter/1 -> Delay/1
  Delay/1 -> Enable at end of barker/1, Reset When Barkers Are Done/1, Barker Even/1, Barker Odd/1
  Vector Concatenate1/1 -> Delay1/1
  Enable at end of barker/1 -> Delay2/1
  Unpack1/1(Out1) -> Delay3/1
  Delay1/1 -> Switch1/1
  Delay2/1 -> Switch1/2
  Delay3/1 -> Switch1/3

== system RxTxFixedPointLibrary/Transmitter HDL/Packet Generation/Random Data ==
  In1 : Inport
  Random Data Gen1 : commseqgen3/PN Sequence Generator  poly='z^10 + z^7 + 1'  ini_sta=[0 0 1 0 0 1 0 0 1 1]  outBitMaskSource=Dialog parameter  shift=0  outVarSiz=off  maxOutSizeMode=Dialog parameter  maxOutSize=[10 1]  Ts=-1  sampPerFrame=1  reset=on  bitPackedOutputs=on  outDataType=double  numPackedBits=2  bitPackDataSigned=off  bitPackedOutDType=Smallest integer
      settings: SourceProductName=Communications System Toolbox
  Unpack : Subsystem
  Out1 : Outport
  wires:
  In1/1 -> Random Data Gen1/1
  Unpack/1(Out1) -> Out1/1
  Random Data Gen1/1 -> Unpack/1(In1)

== system RxTxFixedPointLibrary/Receiver HDL/CRC Check and DMA Pack/DMA Interface/Convert Payload Length To Bytes ==
  In1 : Inport
  Constant : Constant  Value=uint16(32-1)  SampleTime=-1
  Convert To Bytes From Bits : ArithShift  BitShiftNumber=3  BitShiftDirection=Right
  Convert To Uncoded : ArithShift  BitShiftNumber=1  BitShiftDirection=Right
  Data Type Conversion : DataTypeConversion  OutDataTypeStr=uint16
  Remove CRC Length : Sum  Inputs=+-  AccumDataTypeStr=uint16
  packetLengthOut : Outport
  wires:
  Data Type Conversion/1 -> packetLengthOut/1
  Constant/1 -> Remove CRC Length/2
  Convert To Bytes From Bits/1 -> Data Type Conversion/1
  Convert To Uncoded/1 -> Remove CRC Length/1
  Remove CRC Length/1 -> Convert To Bytes From Bits/1
  In1/1 -> Convert To Uncoded/1

== system RxTxFixedPointLibrary/Receiver HDL/Frame Recover/Barker Locate/ABS1 ==
  In1 : Inport
  Add : Sum
  Complex to Real-Imag : ComplexToRealImag
  Product : Product  OutDataTypeStr=int16
  Product1 : Product  OutDataTypeStr=int16
  Out1 : Outport
  wires:
  Add/1 -> Out1/1
  Product1/1 -> Add/2
  Product/1 -> Add/1
  Complex to Real-Imag/1 -> Product/2, Product/1
  Complex to Real-Imag/2 -> Product1/1, Product1/2
  In1/1 -> Complex to Real-Imag/1

== system RxTxFixedPointLibrary/Receiver HDL/Frame Recover/Barker Locate/ABS2 ==
  In1 : Inport
  Add : Sum  SaturateOnIntegerOverflow=on
  Complex to Real-Imag : ComplexToRealImag
  Product : Product  OutDataTypeStr=int16
  Product1 : Product  OutDataTypeStr=int16
  Out1 : Outport
  wires:
  Add/1 -> Out1/1
  Product1/1 -> Add/2
  Product/1 -> Add/1
  Complex to Real-Imag/1 -> Product/2, Product/1
  Complex to Real-Imag/2 -> Product1/1, Product1/2
  In1/1 -> Complex to Real-Imag/1

== system RxTxFixedPointLibrary/Receiver HDL/Frame Recover/Barker Locate/HDL Opt Complex FIR ==
  In1 : Inport
  validIn : Inport  Port=2
  Add : Sum  AccumDataTypeStr=fixdt(1,16,0)
  Discrete FIR Filter HDL Optimized : dsphdlfiltering/Discrete FIR Filter HDL Optimized  Numerator=real(Taps)  Sharing=off  SharingFactor=2  SimulateUsing=Code generation  roundingMode=Floor  overflowMode=off  CoefficientsDataTypeStr=Inherit: Same word length as input  CoefficientsMin=[]  CoefficientsMax=[]  OutputDataTypeStr=fixdt(1,15,0)  OutputMin=[]  OutputMax=[]  ValidInPort=on  ReadyPort=off
      settings: SourceProductName=DSP System Toolbox  SourceProductBaseCode=DS
  Discrete FIR Filter HDL Optimized1 : dsphdlfiltering/Discrete FIR Filter HDL Optimized  Numerator=imag(Taps)  Sharing=off  SharingFactor=2  SimulateUsing=Code generation  roundingMode=Floor  overflowMode=off  CoefficientsDataTypeStr=Inherit: Same word length as input  CoefficientsMin=[]  CoefficientsMax=[]  OutputDataTypeStr=fixdt(1,15,0)  OutputMin=[]  OutputMax=[]  ValidInPort=on  ReadyPort=off
      settings: SourceProductName=DSP System Toolbox  SourceProductBaseCode=DS
  Logical Operator : Logic  AllPortsSameDT=off  OutDataTypeStr=boolean
  Out1 : Outport
  validOut : Outport  Port=2
  wires:
  validIn/1 -> Discrete FIR Filter HDL Optimized/2, Discrete FIR Filter HDL Optimized1/2
  Discrete FIR Filter HDL Optimized1/1 -> Add/2
  Discrete FIR Filter HDL Optimized1/2 -> Logical Operator/2
  Discrete FIR Filter HDL Optimized/2 -> Logical Operator/1
  Logical Operator/1 -> validOut/1
  Add/1 -> Out1/1
  Discrete FIR Filter HDL Optimized/1 -> Add/1
  In1/1 -> Discrete FIR Filter HDL Optimized/1, Discrete FIR Filter HDL Optimized1/1
